simulink model "sim"  (R2018a)
settings: Solver=VariableStepAuto  StartTime=0.0  StopTime=10.0  RelTol=1e-3
values from neighbouring files (symbols this model uses):
  k = 5    [sol.m]
  tao = 2    [sol.m]
  Tm = 0.5    [sol.m]
libraries: fuzblock x1
settings Model: Creator=daniel  LastModifiedBy=daniel

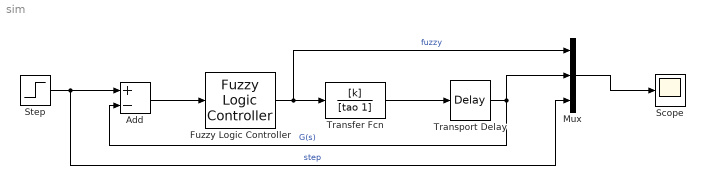
== system sim ==
  Add : Sum  Inputs=+-
  Fuzzy Logic Controller : fuzblock/Fuzzy Logic  Controller  FIS=fcontrol  OutputSampleNumber=101  DataType=double  FuzzifiedInputs=off  RuleFiringStrengths=off  RuleOutputs=off  AggregatedOutputs=off  SimulateUsing=Interpreted execution  OutOfRangeInputValueMessage=warning  NoRuleFiredMessage=warning  EmptyOutputFuzzySetMessage=warning
  Mux : Mux  Inputs=3
  Scope : Scope
  Step : Step  Time=0  SampleTime=0
  Transfer Fcn : TransferFcn  Numerator=[k]  Denominator=[tao 1]
  Transport Delay : TransportDelay  DelayTime=Tm
  wires:
  Transfer Fcn/1 -> Transport Delay/1
  Transport Delay/1 -> Mux/2, Add/2  "G(s)"
  Mux/1 -> Scope/1
  Fuzzy Logic Controller/1 -> Mux/1, Transfer Fcn/1  "fuzzy"
  Step/1 -> Mux/3, Add/1  "step"
  Add/1 -> Fuzzy Logic Controller/1
